simulink subsystem "Soma"  (R2023b)
settings: Solver=VariableStepAuto  StartTime=0.0  StopTime=10.0  RelTol=1e-3
undefined symbols (not defined in the file): EgoCar1_params, Ts
libraries: autolibshared x1, simulink_extras x1
settings Model: Creator=victor  LastModifiedBy=Victor

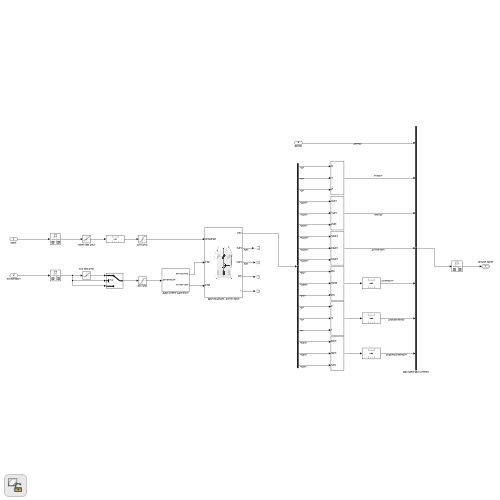
[thumbnail: Simulink's stored preview of the top-level diagram]
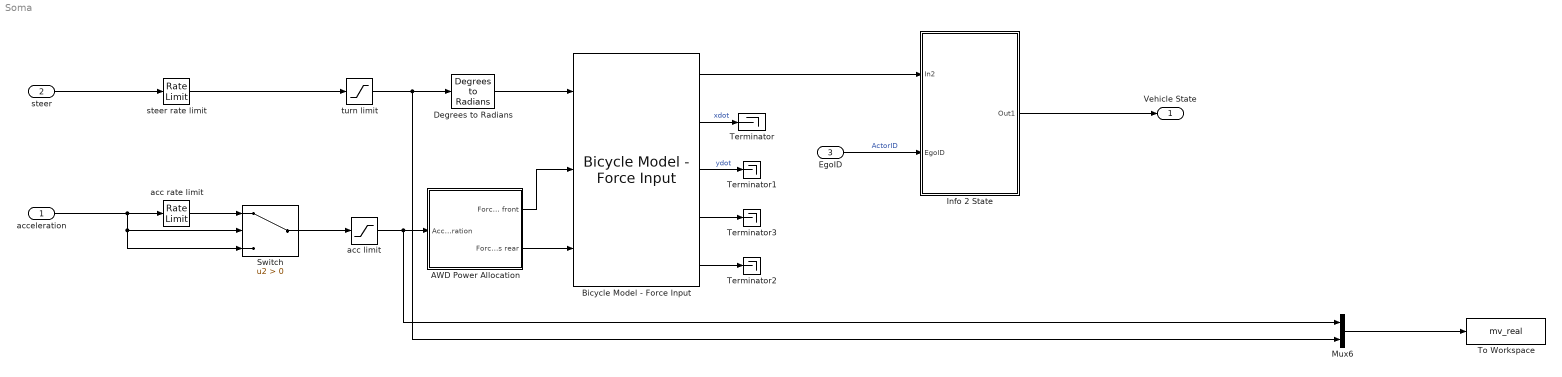
== system Soma ==
  acceleration : Inport  Unit=m/s^2  PortDimensions=1  SampleTime=Ts
  steer : Inport  Port=2  Unit=deg  PortDimensions=1  SampleTime=Ts
  EgoID : Inport  Port=3
  AWD Power Allocation : Subsystem  TreatAsAtomicUnit=on
  Bicycle Model - Force Input : autolibshared/Bicycle Model - Force Input  trackMode=Single (bicycle)  inputMode=External longitudinal forces  frontSteerMode=on  rearSteerMode=off  windMode=off  muMode=off  extFMode=off  extMMode=off  aMode=3  NF=2  NR=2  m=EgoCar1_params.Dynamics.m  a=EgoCar1_params.Dynamics.lf  b=EgoCar1_params.Dynamics.lr  h=0.35  X_o=EgoCar1_params.State.Position(1)  xdot_o=EgoCar1_params.State.Velocity(1)  CalphaMode=off  sigmaMode=on  w=[1.4,1.4]  Cy_f=EgoCar1_params.Dynamics.Cf  Cy_r=EgoCar1_params.Dynamics.Cr  sigma_f=.1  sigma_r=.1  alpha_f_brk=[-.1 .1]  Cy_f_data=[-9e3 9e3]  alpha_r_brk=[-.1 .1]  Cy_r_data=[-9e3 9e3]  Y_o=EgoCar1_params.State.Position(2)  ydot_o=EgoCar1_params.State.Velocity(2)  Izz=EgoCar1_params.Dynamics.Iz  psi_o=EgoCar1_params.State.Orientation(3)  r_o=EgoCar1_params.State.AngularVelocity(3)  Af=0  Cd=.3  Cl=.1  Cpm=.1  beta_w=[0:0.01:0.3]  Cs=[0:0.03:0.9]  Cym=[0:0.01:0.3]  Pabs=101325  Tair=273  g=9.81  mu=1  xdot_tol=.01  Fznom=EgoCar1_params.Dynamics.m*9.81/2  Fxtire_sat=1e6  Fytire_sat=1e6  longOff=0  latOff=0  vertOff=0
      settings: LibrarySourceBlock=drivingscenarioandsensors/Bicycle Model - Force Input
  Degrees to Radians : simulink_extras/Transformations/Degrees to Radians
  Info 2 State : Subsystem  TreatAsAtomicUnit=on
  Mux6 : Mux  Inputs=2
  Switch : Switch  Criteria=u2 > Threshold  SaturateOnIntegerOverflow=off  InputSameDT=off
  Terminator{,1..3} (4 alike) : Terminator
  To Workspace : ToWorkspace  VariableName=mv_real  SaveFormat=Timeseries  SampleTime=-1
  acc limit : Saturate  UpperLimit=EgoCar1_params.Limits.accMAX*1.5  LowerLimit=-EgoCar1_params.Limits.brakeMAX*1.5
  acc rate limit : RateLimiter  RisingSlewLimit=EgoCar1_params.Limits.jerkMAX*1.5  FallingSlewLimit=-EgoCar1_params.Limits.jerkMAX*1.5  SampleTimeMode=inherited
  steer rate limit : RateLimiter  RisingSlewLimit=EgoCar1_params.Limits.turnAngleRateMAX*1.5  FallingSlewLimit=-EgoCar1_params.Limits.turnAngleRateMAX*1.5  SampleTimeMode=inherited
  turn limit : Saturate  UpperLimit=EgoCar1_params.Limits.turnAngleMAX*1.5  LowerLimit=-EgoCar1_params.Limits.turnAngleMAX*1.5
  Vehicle State : Outport  OutDataTypeStr=Bus: BusEgoVehicleState  SampleTime=Ts
  wires:
  Bicycle Model - Force Input/4 -> Terminator3/1
  acc limit/1 -> AWD Power Allocation/1(Acceleration), Mux6/1
  Degrees to Radians/1 -> Bicycle Model - Force Input/1
  Bicycle Model - Force Input/5 -> Terminator2/1
  acceleration/1 -> Switch/3, Switch/2, acc rate limit/1
  steer/1 -> steer rate limit/1
  Bicycle Model - Force Input/2 -> Terminator/1  "xdot"
  AWD Power Allocation/1(Forces front) -> Bicycle Model - Force Input/2
  Switch/1 -> acc limit/1
  AWD Power Allocation/2(Forces rear) -> Bicycle Model - Force Input/3
  Bicycle Model - Force Input/3 -> Terminator1/1  "ydot"
  acc rate limit/1 -> Switch/1
  steer rate limit/1 -> turn limit/1
  turn limit/1 -> Degrees to Radians/1, Mux6/2
  Mux6/1 -> To Workspace/1
  EgoID/1 -> Info 2 State/2(EgoID)  "ActorID"
  Bicycle Model - Force Input/1 -> Info 2 State/1(In2)
  Info 2 State/1(Out1) -> Vehicle State/1

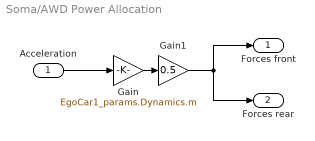
== system Soma/AWD Power Allocation ==
  Acceleration : Inport
  Gain : Gain  Gain=EgoCar1_params.Dynamics.m
  Gain1 : Gain  Gain=0.5
  Forces front : Outport  VectorParamsAs1DForOutWhenUnconnected=off
  Forces rear : Outport  Port=2  VectorParamsAs1DForOutWhenUnconnected=off
  wires:
  Gain/1 -> Gain1/1
  Gain1/1 -> Forces front/1, Forces rear/1
  Acceleration/1 -> Gain/1

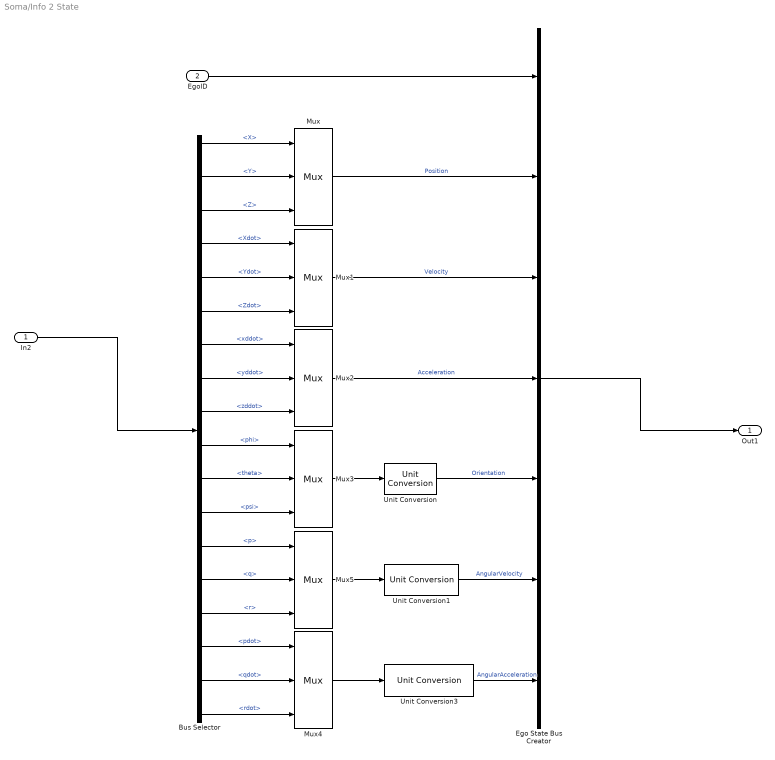
== system Soma/Info 2 State ==
  In2 : Inport
  EgoID : Inport  Port=2
  Bus Selector : BusSelector  OutputSignals=InertFrm.Cg.Disp.X,InertFrm.Cg.Disp.Y,InertFrm.Cg.Disp.Z,InertFrm.Cg.Vel.Xdot,InertFrm.Cg.Vel.Ydot,InertFrm.Cg.Vel.Zdot,BdyFrm.Cg.Acc.xddot,BdyFrm.Cg.Acc.yddot,BdyFrm.Cg.Acc.zddot,InertFrm.Cg.Ang.phi,InertFrm.Cg.Ang.theta,InertFrm.Cg.Ang.psi,BdyFrm.Cg.AngVel.p,BdyFrm.Cg.AngVel.q,BdyFrm.Cg.AngVel.r,BdyFrm.Cg.AngAcc.pdot,BdyFrm.Cg.AngAcc.qdot,BdyFrm.Cg.AngAcc.rdot
  Ego State Bus Creator : BusCreator  Inputs=7  OutDataTypeStr=Bus: BusEgoVehicleState  NonVirtualBus=on
  Mux{,1..5} (6 alike) : Mux  Inputs=3
      settings: DisplayOption=signals
  Unit Conversion : UnitConversion  OutputType=Inherit: Inherit via back propagation
  Unit Conversion1 : UnitConversion  OutputType=Inherit: Inherit via back propagation
  Unit Conversion3 : UnitConversion  OutputType=Inherit: Inherit via back propagation
  Out1 : Outport
  wires:
  Ego State Bus Creator/1 -> Out1/1
  In2/1 -> Bus Selector/1
  Unit Conversion/1 -> Ego State Bus Creator/5  "Orientation"
  Bus Selector/4 -> Mux1/1  "<Xdot>"
  Bus Selector/2 -> Mux/2  "<Y>"
  Unit Conversion3/1 -> Ego State Bus Creator/7  "AngularAcceleration"
  EgoID/1 -> Ego State Bus Creator/1
  Bus Selector/8 -> Mux2/2  "<yddot>"
  Bus Selector/6 -> Mux1/3  "<Zdot>"
  Bus Selector/12 -> Mux3/3  "<psi>"
  Bus Selector/14 -> Mux5/2  "<q>"
  Bus Selector/9 -> Mux2/3  "<zddot>"
  Mux2/1 -> Ego State Bus Creator/4  "Acceleration"
  Bus Selector/13 -> Mux5/1  "<p>"
  Mux3/1 -> Unit Conversion/1
  Mux/1 -> Ego State Bus Creator/2  "Position"
  Bus Selector/11 -> Mux3/2  "<theta>"
  Bus Selector/10 -> Mux3/1  "<phi>"
  Bus Selector/5 -> Mux1/2  "<Ydot>"
  Unit Conversion1/1 -> Ego State Bus Creator/6  "AngularVelocity"
  Bus Selector/7 -> Mux2/1  "<xddot>"
  Bus Selector/18 -> Mux4/3  "<rdot>"
  Mux5/1 -> Unit Conversion1/1
  Mux1/1 -> Ego State Bus Creator/3  "Velocity"
  Bus Selector/15 -> Mux5/3  "<r>"
  Bus Selector/16 -> Mux4/1  "<pdot>"
  Bus Selector/17 -> Mux4/2  "<qdot>"
  Mux4/1 -> Unit Conversion3/1
  Bus Selector/1 -> Mux/1  "<X>"
  Bus Selector/3 -> Mux/3  "<Z>"
